simulink model "cruise_from_template"  (R2021a)
settings: Solver=ode3  StartTime=0.0  StopTime=60  FixedStep=1/120  RelTol=1e-5
model workspace (MATLAB code in the model file + MAT data in the model file):
  aeroCoeff.Cl0 = 0
  aeroCoeff.Cl_beta = -0.0325103964148
  aeroCoeff.Cl_da = -0.11683362461
  aeroCoeff.Cl_da_alpha = 0
  aeroCoeff.Cl_dr = 0.175731928031
  aeroCoeff.Cl_p = -0.836747044856
  aeroCoeff.Cl_r = 0.21079983888
  aeroCoeff.Cm0 = 0
  aeroCoeff.Cm_alpha = 2.67718247065
  aeroCoeff.Cm_alpha2 = 0
  aeroCoeff.Cm_beta2 = 0
  aeroCoeff.Cm_de = 2.06131250249
  aeroCoeff.Cm_df = 0
  aeroCoeff.Cm_q = -44.2196099405
  aeroCoeff.Cm_r = 0
  aeroCoeff.Cn0 = 0
  aeroCoeff.Cn_beta = 0.049110167229
  aeroCoeff.Cn_beta3 = 0
  aeroCoeff.Cn_da = 0.0191607144361
  aeroCoeff.Cn_dr = -0.388239776666
  aeroCoeff.Cn_p = -0.0358992823949
  aeroCoeff.Cn_q = 0.1595
  aeroCoeff.Cn_r = -0.0711145772129
  aeroCoeff.Cx0 = 0
  aeroCoeff.Cx_alpha = 0.609676812174
  aeroCoeff.Cx_alpha2 = 0
  aeroCoeff.Cx_alpha3 = 0
  aeroCoeff.Cx_df = 0
  aeroCoeff.Cx_df_alpha = 0
  aeroCoeff.Cx_dr = 0
  aeroCoeff.Cx_q = 0
  aeroCoeff.Cx_de = 0
  aeroCoeff.Cy0 = 0
  aeroCoeff.Cy_beta = -0.163321495037
  aeroCoeff.Cy_da = 0
  aeroCoeff.Cy_dr = 0.921751820421
  aeroCoeff.Cy_dr_alpha = 0
  aeroCoeff.Cy_p = -0.0243192462004
  aeroCoeff.Cy_r = 0.137581286748
  aeroCoeff.Cz0 = -0.82
  aeroCoeff.Cz_alpha = -3.9329056742
  aeroCoeff.Cz_alpha3 = 0
  aeroCoeff.Cz_de = -0.761136778285
  aeroCoeff.Cz_de_beta = 0
  aeroCoeff.Cz_df = 0
  aeroCoeff.Cz_df_alpha = 0
  aeroCoeff.Cz_q = 0.451102723983
  aeroCoeff.V0 = 64.72
  aeroCoeff.Cx_u = -0.223869966065
  aeroCoeff.Cz_u = -0.031521374419
  aeroCoeff.Cm_u = -0.00247698437476
  aeroCoeff.Cx_adot = 0
  aeroCoeff.Cz_adot = -5.62744914371
  aeroCoeff.Cm_adot = -19.0854006767
  environment.EarthRefAlt = 0
  initCond.x0 = [0 0 -1000]
  initCond.v0 = [64.72 0 0]
  initCond.euler0 = [0 0 0]
  initCond.w0 = [0 0 0]
  inputs0.time = 0
  inputs0.signals(1).dimensions = 1
  inputs0.signals(1).values = -0.104711430294
  inputs0.signals(2).dimensions = 1
  inputs0.signals(2).values = -0.0698725229544
  inputs0.signals(3).dimensions = 1
  inputs0.signals(3).values = -0.000215042330254
  states0.time = 0
  states0.signals(1).values = [0 0 -1000]
  states0.signals(1).dimensions = 3
  states0.signals(1).label = 'CSTATE'
  states0.signals(1).blockName = 'asb6DOFAirframeTemplate/6DOF EOM/6DOF (Euler Angles)/xe,ye,ze'
  states0.signals(1).stateName = ''
  states0.signals(1).inReferencedModel = 0
  states0.signals(1).sampleTime = [0 0]
  states0.signals(2).values = [0.128665353089 0.259337659946 -0.178947917154]
  states0.signals(2).dimensions = 3
  states0.signals(2).label = 'CSTATE'
  states0.signals(2).blockName = 'asb6DOFAirframeTemplate/6DOF EOM/6DOF (Euler Angles)/Calculate DCM &
    | Euler Angles/phi
    | theta
    | psi'
  states0.signals(2).stateName = ''
  states0.signals(2).inReferencedModel = 0
  states0.signals(2).sampleTime = [0 0]
  states0.signals(3).values = [36.9119692666 8.10720863264 8.82591882596]
  states0.signals(3).dimensions = 3
  states0.signals(3).label = 'CSTATE'
  states0.signals(3).blockName = 'asb6DOFAirframeTemplate/6DOF EOM/6DOF (Euler Angles)/ub,vb,wb'
  states0.signals(3).stateName = ''
  states0.signals(3).inReferencedModel = 0
  states0.signals(3).sampleTime = [0 0]
  states0.signals(4).values = [0 0 0]
  states0.signals(4).dimensions = 3
  states0.signals(4).label = 'CSTATE'
  states0.signals(4).blockName = 'asb6DOFAirframeTemplate/6DOF EOM/6DOF (Euler Angles)/p,q,r '
  states0.signals(4).stateName = ''
  states0.signals(4).inReferencedModel = 0
  states0.signals(4).sampleTime = [0 0]
  states0.signals(5).values = [0 0]
  states0.signals(5).dimensions = 2
  states0.signals(5).label = 'CSTATE'
  states0.signals(5).blockName = 'asb6DOFAirframeTemplate/Environment Model/Dryden Wind Turbulence Model 
    | (Continuous (+q +r))/Filters on velocities/Hwgw(s)/wg_p1'
  states0.signals(5).stateName = ''
  states0.signals(5).inReferencedModel = 0
  states0.signals(5).sampleTime = [0 0]
  states0.signals(6).values = [0 0]
  states0.signals(6).dimensions = 2
  states0.signals(6).label = 'CSTATE'
  states0.signals(6).blockName = 'asb6DOFAirframeTemplate/Environment Model/Dryden Wind Turbulence Model 
    | (Continuous (+q +r))/Filters on velocities/Hwgw(s)/wg_p2'
  states0.signals(6).stateName = ''
  states0.signals(6).inReferencedModel = 0
  states0.signals(6).sampleTime = [0 0]
  states0.signals(7).values = [0 0]
  states0.signals(7).dimensions = 2
  states0.signals(7).label = 'CSTATE'
  states0.signals(7).blockName = 'asb6DOFAirframeTemplate/Environment Model/Dryden Wind Turbulence Model 
    | (Continuous (+q +r))/Filters on velocities/Hvgw(s)/vg_p1'
  states0.signals(7).stateName = ''
  states0.signals(7).inReferencedModel = 0
  states0.signals(7).sampleTime = [0 0]
  states0.signals(8).values = [0 0]
  states0.signals(8).dimensions = 2
  states0.signals(8).label = 'CSTATE'
  states0.signals(8).blockName = 'asb6DOFAirframeTemplate/Environment Model/Dryden Wind Turbulence Model 
    | (Continuous (+q +r))/Filters on velocities/Hvgw(s)/vgw_p2'
  states0.signals(8).stateName = ''
  states0.signals(8).inReferencedModel = 0
  states0.signals(8).sampleTime = [0 0]
  states0.signals(9).values = [0 0]
  states0.signals(9).dimensions = 2
  states0.signals(9).label = 'CSTATE'
  states0.signals(9).blockName = 'asb6DOFAirframeTemplate/Environment Model/Dryden Wind Turbulence Model 
    | (Continuous (+q +r))/Filters on velocities/Hugw(s)/ug_p'
  states0.signals(9).stateName = ''
  states0.signals(9).inReferencedModel = 0
  states0.signals(9).sampleTime = [0 0]
  states0.signals(10).values = [0 0]
  states0.signals(10).dimensions = 2
  states0.signals(10).label = 'CSTATE'
  states0.signals(10).blockName = 'asb6DOFAirframeTemplate/Environment Model/Dryden Wind Turbulence Model 
    | (Continuous (+q +r))/Filters on angular rates/Hrgw/rgw_p'
  states0.signals(10).stateName = ''
  states0.signals(10).inReferencedModel = 0
  states0.signals(10).sampleTime = [0 0]
  states0.signals(11).values = [0 0]
  states0.signals(11).dimensions = 2
  states0.signals(11).label = 'CSTATE'
  states0.signals(11).blockName = 'asb6DOFAirframeTemplate/Environment Model/Dryden Wind Turbulence Model 
    | (Continuous (+q +r))/Filters on angular rates/Hqgw/qgw_p'
  states0.signals(11).stateName = ''
  states0.signals(11).inReferencedModel = 0
  states0.signals(11).sampleTime = [0 0]
  states0.signals(12).values = [0 0]
  states0.signals(12).dimensions = 2
  states0.signals(12).label = 'CSTATE'
  states0.signals(12).blockName = 'asb6DOFAirframeTemplate/Environment Model/Dryden Wind Turbulence Model 
    | (Continuous (+q +r))/Filters on angular rates/Hpgw/pgw_p'
  states0.signals(12).stateName = ''
  states0.signals(12).inReferencedModel = 0
  states0.signals(12).sampleTime = [0 0]
  vehicle.Sref = 16.834
  vehicle.cbar = 1.0141
  vehicle.bref = 8.704
  vehicle.CG = [0 0 0]
  vehicle.CP = [0 0 0]
  vehicle.inertia = [13609.1339893  0  146.582252166; 0  23776.5214  0; -146.582252166  0  34194.8393722]
  vehicle.acMass = 2950
  vehicle.Thrust = 2300
  vehicle.aileron_max = 0.523598775598
  vehicle.aileron_min = -0.523598775598
  vehicle.elevator_max = 0.305432619099
  vehicle.elevator_min = -0.305432619099
  vehicle.rudder_max = 0.436332312999
  vehicle.rudder_min = -0.436332312999
  other statements: initialize6DOFSkyHogg;
undefined symbols (not defined in the file): p, q, r
libraries: aerolibasang x3, shared6dof x1, aerolibadyn x1, aerolibatmos2 x1
settings Model: Creator=jakob  LastModifiedBy=jakob
settings SolverCC: AlgebraicLoopSolver=TrustRegion  AutoInsertRateTranBlk=on  InsertRTBMode=Never (minimum delay)  MinimalZcImpactIntegration=on
settings DataIOCC: ExternalInput=inputs0  InitialState=states0  SaveFormat=Array  SaveOutput=off
settings OptimizationCC: EnhancedBackFolding=on  StrengthReduction=on  InitFltsAndDblsToZero=on  DifferentSizesBufferReuse=on
settings DebuggingCC: WriteAfterWriteMsg=DisableAll  AlgebraicLoopMsg=none  FcnCallInpInsideContextMsg=warning  UnconnectedInputMsg=none  UnconnectedOutputMsg=none  UnconnectedLineMsg=none  UniqueDataStoreMsg=error  RootOutportRequireBusObject=none  StateNameClashWarn=warning  StrictBusMsg=ErrorOnBusTreatedAsVector  SFUnexpectedBacktrackingDiag=warning  SFNoUnconditionalDefaultTransitionDiag=warning  SFExecutionAtInitializationDiag=none  SFMachineParentedDataDiag=warning  ArithmeticOperatorsInVariantConditions=warning
settings ModelReferenceCC: PropagateSignalLabelsOutOfModel=off
settings SFSimCC: SimUseLocalCustomCode=off
settings RTWCC: RTWUseLocalCustomCode=off
settings CodeAppCC: StateflowObjectComments=on

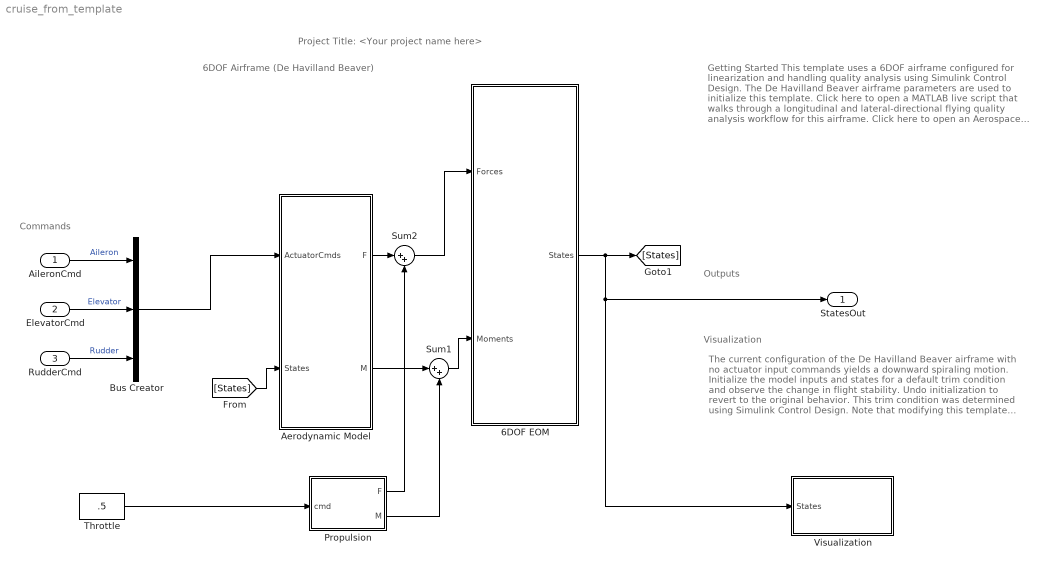
== system cruise_from_template ==
  note: Project Title: <Your project name here>
  note: 6DOF Airframe (De Havilland Beaver)
  note: Commands
  note: The current configuration of the De Havilland Beaver airframe with no actuator input commands yields a downward spiraling motion. Initialize the model inputs and states for a default trim condition and observe the change in flight stability. Undo initialization to revert to the original behavior. This trim condition was determined using Simulink Control Design. Note that modifying this template model may invalidate the default trim condition.
  note: Visualization
  note: Outputs
  note: Getting Started
      | This template uses a 6DOF airframe configured for linearization and handling quality analysis using Simulink Control Design. The De Havilland Beaver airframe parameters are used to initialize this template.
      |
      | Click here to open a MATLAB live script that walks through a longitudinal and lateral-directional flying quality analysis workflow for this airframe.
      |
      | Click here to open an Aerospace Blockset Flight Control Analysis template that can be customized to perform flying quality analysis on your airframe model.
  AileronCmd : Inport
  ElevatorCmd : Inport  Port=2
  RudderCmd : Inport  Port=3
  6DOF EOM : Subsystem  VariantControl=eom3DOF
  Aerodynamic Model : Subsystem  VariantControl=aeroCONST
  Bus Creator : BusCreator  Inputs=3
  Propulsion : Subsystem
      settings: RTWSystemCode=Inline
  Sum1 : Sum  Inputs=|++  InputSameDT=on  SaturateOnIntegerOverflow=on  OutDataTypeStr=Inherit: Same as first input
  Sum2 : Sum  Inputs=|++  InputSameDT=on  SaturateOnIntegerOverflow=on  OutDataTypeStr=Inherit: Same as first input
  Throttle : Constant  Value=.5
  Visualization : Subsystem
  StatesOut : Outport  OutDataTypeStr=double  VectorParamsAs1DForOutWhenUnconnected=off
  wires:
  AileronCmd/1 -> Bus Creator/1  "Aileron"
  ElevatorCmd/1 -> Bus Creator/2  "Elevator"
  RudderCmd/1 -> Bus Creator/3  "Rudder"
  [States] -> Aerodynamic Model/2(States)
  6DOF EOM/1(States) -> [States], StatesOut/1, Visualization/1(States)
  Sum2/1 -> 6DOF EOM/1(Forces)
  Propulsion/2(M) -> Sum1/2
  Propulsion/1(F) -> Sum2/2
  Throttle/1 -> Propulsion/1(cmd)
  Sum1/1 -> 6DOF EOM/2(Moments)
  Aerodynamic Model/1(F) -> Sum2/1
  Aerodynamic Model/2(M) -> Sum1/1
  Bus Creator/1 -> Aerodynamic Model/1(ActuatorCmds)

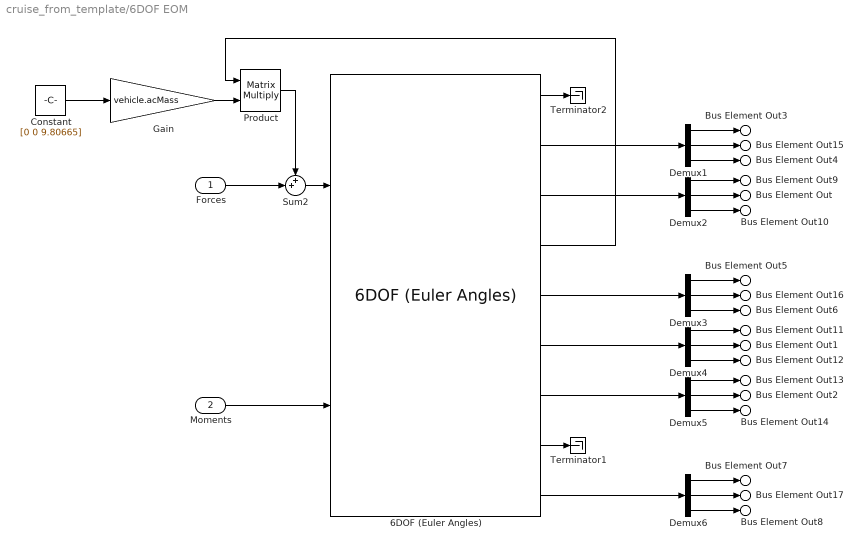
== system cruise_from_template/6DOF EOM ==
  Forces : Inport
  Moments : Inport  Port=2
  6DOF (Euler Angles) : shared6dof/6DOF (Euler Angles)  units=Metric (MKS)  mtype=Fixed  rep=Euler Angles  xme_0=initCond.x0  Vm_0=initCond.v0  eul_0=initCond.euler0  pm_0=initCond.w0  mass_0=vehicle.acMass  mass_e=0.5  mass_f=2.0  inertia=vehicle.inertia  inertia_e=eye(3)  inertia_f=2*eye(3)  k_quat=1.0  vre_flag=on  abi_flag=on  aMode=0  xme_statename={'Xe', 'Ye', 'Ze'}  Vm_statename={'Ubody', 'Vbody', 'Wbody'}  eul_statename={'phi', 'theta', 'psi'}  quat_statename={'qr', 'qi', 'qj','qk'}  pm_statename={'p', 'q', 'r'}  mass_statename=''
      settings: SourceProductBaseCode=AE,PW,DR,MT,UV,VE
  Constant : Constant  Value=[0 0 9.80665]
  Demux{1..6} (6 alike) : Demux  Outputs=3
  Gain : Gain  Gain=vehicle.acMass
  Product : Product  Multiplication=Matrix(*)
  Sum2 : Sum  Inputs=++|  InputSameDT=on  SaturateOnIntegerOverflow=on  OutDataTypeStr=Inherit: Same as first input
  Terminator1 : Terminator
  Terminator2 : Terminator
  Bus Element Out3 : Outport  VectorParamsAs1DForOutWhenUnconnected=off  PortName=States  Element=Xe
  Bus Element Out4 : Outport  VectorParamsAs1DForOutWhenUnconnected=off  PortName=States  Element=Ze
  Bus Element Out : Outport  VectorParamsAs1DForOutWhenUnconnected=off  PortName=States  Element=theta
  Bus Element Out5 : Outport  VectorParamsAs1DForOutWhenUnconnected=off  PortName=States  Element=u
  Bus Element Out6 : Outport  VectorParamsAs1DForOutWhenUnconnected=off  PortName=States  Element=w
  Bus Element Out1 : Outport  VectorParamsAs1DForOutWhenUnconnected=off  PortName=States  Element=q
  Bus Element Out2 : Outport  VectorParamsAs1DForOutWhenUnconnected=off  PortName=States  Element=q_dot
  Bus Element Out7 : Outport  VectorParamsAs1DForOutWhenUnconnected=off  PortName=States  Element=Axe
  Bus Element Out8 : Outport  VectorParamsAs1DForOutWhenUnconnected=off  PortName=States  Element=Aze
  Bus Element Out15 : Outport  VectorParamsAs1DForOutWhenUnconnected=off  PortName=States  Element=Ye
  Bus Element Out9 : Outport  VectorParamsAs1DForOutWhenUnconnected=off  PortName=States  Element=phi
  Bus Element Out10 : Outport  VectorParamsAs1DForOutWhenUnconnected=off  PortName=States  Element=psi
  Bus Element Out16 : Outport  VectorParamsAs1DForOutWhenUnconnected=off  PortName=States  Element=v
  Bus Element Out11 : Outport  VectorParamsAs1DForOutWhenUnconnected=off  PortName=States  Element=p
  Bus Element Out12 : Outport  VectorParamsAs1DForOutWhenUnconnected=off  PortName=States  Element=r
  Bus Element Out13 : Outport  VectorParamsAs1DForOutWhenUnconnected=off  PortName=States  Element=p_dot
  Bus Element Out14 : Outport  VectorParamsAs1DForOutWhenUnconnected=off  PortName=States  Element=r_dot
  Bus Element Out17 : Outport  VectorParamsAs1DForOutWhenUnconnected=off  PortName=States  Element=Aye
  wires:
  6DOF (Euler Angles)/2 -> Demux1/1
  6DOF (Euler Angles)/4 -> Product/1
  6DOF (Euler Angles)/1 -> Terminator2/1
  Demux6/2 -> Bus Element Out17/1
  Demux6/3 -> Bus Element Out8/1
  Demux6/1 -> Bus Element Out7/1
  6DOF (Euler Angles)/9 -> Demux6/1
  6DOF (Euler Angles)/7 -> Demux5/1
  Demux5/3 -> Bus Element Out14/1
  Demux5/2 -> Bus Element Out2/1
  Demux5/1 -> Bus Element Out13/1
  6DOF (Euler Angles)/6 -> Demux4/1
  Demux4/3 -> Bus Element Out12/1
  Demux4/2 -> Bus Element Out1/1
  Demux4/1 -> Bus Element Out11/1
  Demux3/3 -> Bus Element Out6/1
  Demux3/2 -> Bus Element Out16/1
  Demux3/1 -> Bus Element Out5/1
  6DOF (Euler Angles)/5 -> Demux3/1
  Demux2/3 -> Bus Element Out10/1
  Demux2/2 -> Bus Element Out/1
  Demux2/1 -> Bus Element Out9/1
  Demux1/1 -> Bus Element Out3/1
  Demux1/3 -> Bus Element Out4/1
  Demux1/2 -> Bus Element Out15/1
  Gain/1 -> Product/2
  6DOF (Euler Angles)/3 -> Demux2/1
  Moments/1 -> 6DOF (Euler Angles)/2
  Forces/1 -> Sum2/2
  Sum2/1 -> 6DOF (Euler Angles)/1
  Product/1 -> Sum2/1
  6DOF (Euler Angles)/8 -> Terminator1/1
  Constant/1 -> Gain/1

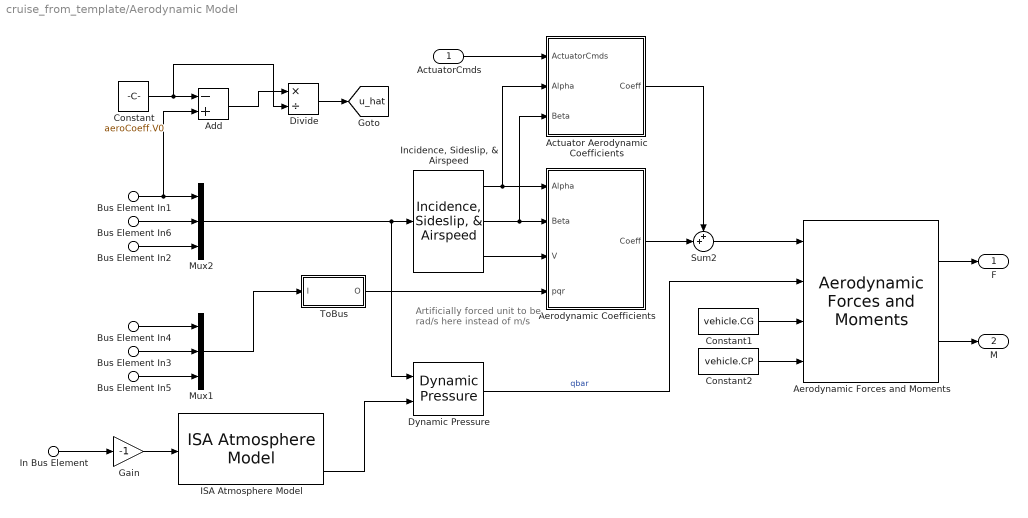
== system cruise_from_template/Aerodynamic Model ==
  note: Artificially forced unit to be
      | rad/s here instead of m/s
  ActuatorCmds : Inport
  Bus Element In1 : Inport  Port=2  PortName=States  Element=u
  Bus Element In2 : Inport  Port=2  PortName=States  Element=w
  Bus Element In3 : Inport  Port=2  PortName=States  Element=q
  Bus Element In6 : Inport  Port=2  PortName=States  Element=v
  Bus Element In4 : Inport  Port=2  PortName=States  Element=p
  Bus Element In5 : Inport  Port=2  PortName=States  Element=r
  In Bus Element : Inport  Port=2  PortName=States  Element=Ze
  Actuator Aerodynamic Coefficients : Subsystem
  Add : Sum  Inputs=-+
  Aerodynamic Coefficients : Subsystem
  Aerodynamic Forces and Moments : aerolibadyn/Aerodynamic Forces and Moments   inputAxes=Body  outputForceAxes=Body  outputMomentAxes=Body  S=vehicle.Sref  b=vehicle.bref  cbar=vehicle.cbar
  Constant : Constant  Value=aeroCoeff.V0
  Constant1 : Constant  Value=vehicle.CG
  Constant2 : Constant  Value=vehicle.CP
  Divide : Product  Inputs=*/
  Dynamic Pressure : aerolibasang/Dynamic Pressure
  Gain : Gain  Gain=-1
  ISA Atmosphere Model : aerolibatmos2/ISA Atmosphere Model  custom=off  g=9.80665  gamma=1.4  R=287.0531  L=0.0065  h_trop=11000  h_strat=20000  rho0=1.225  P0=101325  T0=288.15  h0=0
  "Incidence, Sideslip, & Airspeed" : aerolibasang/Incidence, Sideslip, & Airspeed
  Mux1 : Mux  Inputs=3
  Mux2 : Mux  Inputs=3
  Sum2 : Sum  Inputs=++|
  ToBus : Subsystem
  F : Outport  Unit=N  VectorParamsAs1DForOutWhenUnconnected=off
  M : Outport  Port=2  Unit=N*m  VectorParamsAs1DForOutWhenUnconnected=off
  tag scope: u_hat=global
  wires:
  ActuatorCmds/1 -> Actuator Aerodynamic Coefficients/1(ActuatorCmds)
  Bus Element In5/1 -> Mux1/3
  Bus Element In3/1 -> Mux1/2
  Bus Element In4/1 -> Mux1/1
  Actuator Aerodynamic Coefficients/1(Coeff) -> Sum2/1
  Aerodynamic Coefficients/1(Coeff) -> Sum2/2
  ToBus/1(O) -> Aerodynamic Coefficients/4(pqr)
  Mux2/1 -> Dynamic Pressure/1, "Incidence, Sideslip, & Airspeed"/1
  Dynamic Pressure/1 -> Aerodynamic Forces and Moments/2  "qbar"
  "Incidence, Sideslip, & Airspeed"/3 -> Aerodynamic Coefficients/3(V)
  "Incidence, Sideslip, & Airspeed"/2 -> Aerodynamic Coefficients/2(Beta), Actuator Aerodynamic Coefficients/3(Beta)
  Aerodynamic Forces and Moments/2 -> M/1
  Aerodynamic Forces and Moments/1 -> F/1
  Constant2/1 -> Aerodynamic Forces and Moments/4
  Constant1/1 -> Aerodynamic Forces and Moments/3
  Sum2/1 -> Aerodynamic Forces and Moments/1
  Bus Element In1/1 -> Add/2, Mux2/1
  Bus Element In6/1 -> Mux2/2
  Bus Element In2/1 -> Mux2/3
  "Incidence, Sideslip, & Airspeed"/1 -> Actuator Aerodynamic Coefficients/2(Alpha), Aerodynamic Coefficients/1(Alpha)
  Mux1/1 -> ToBus/1(I)
  ISA Atmosphere Model/4 -> Dynamic Pressure/2
  In Bus Element/1 -> Gain/1
  Gain/1 -> ISA Atmosphere Model/1
  Divide/1 -> [u_hat]
  Constant/1 -> Divide/2, Add/1
  Add/1 -> Divide/1

== system cruise_from_template/Propulsion ==
  cmd : Inport
  Mux : Mux  Inputs=[1 2]
  ThrustX : Lookup_n-D  NumberOfTableDimensions=1  LookupTableObject=''  BreakpointsForDimension1=(1/6)*(3+([-3:3]))  IndexSearchMethod=Linear search  BeginIndexSearchUsingPreviousIndexResult=on  Table=vehicle.Thrust*(1+tanh([-3:3]))  ExtrapMethod=Clip  InputSameDT=on
  ThrustYZ : Constant  Value=[0 0]'  SampleTime=-1
  Thrust_M1 : Constant  Value=[0 0 0]'  SampleTime=-1
  F : Outport  Unit=N  VectorParamsAs1DForOutWhenUnconnected=off
  M : Outport  Port=2  Unit=N*m  VectorParamsAs1DForOutWhenUnconnected=off
  wires:
  Thrust_M1/1 -> M/1
  ThrustX/1 -> Mux/1
  ThrustYZ/1 -> Mux/2
  Mux/1 -> F/1
  cmd/1 -> ThrustX/1

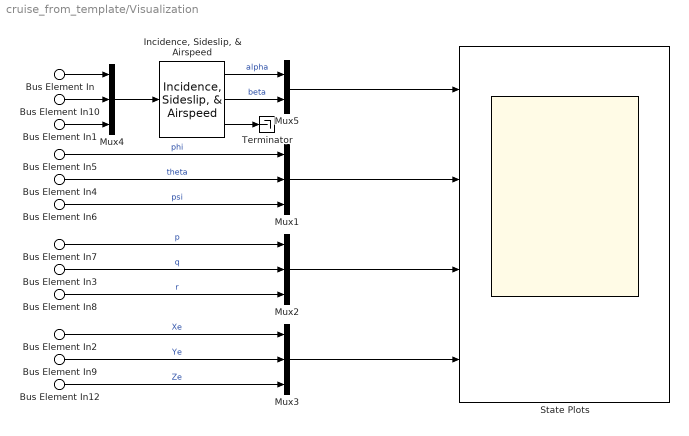
== system cruise_from_template/Visualization ==
  Bus Element In : Inport  PortName=States  Element=u
  Bus Element In1 : Inport  PortName=States  Element=w
  Bus Element In3 : Inport  PortName=States  Element=q
  Bus Element In4 : Inport  PortName=States  Element=theta
  Bus Element In12 : Inport  PortName=States  Element=Ze
  Bus Element In2 : Inport  PortName=States  Element=Xe
  Bus Element In10 : Inport  PortName=States  Element=v
  Bus Element In5 : Inport  PortName=States  Element=phi
  Bus Element In6 : Inport  PortName=States  Element=psi
  Bus Element In7 : Inport  PortName=States  Element=p
  Bus Element In8 : Inport  PortName=States  Element=r
  Bus Element In9 : Inport  PortName=States  Element=Ye
  "Incidence, Sideslip, & Airspeed" : aerolibasang/Incidence, Sideslip, & Airspeed
  Mux{1..4} (4 alike) : Mux  Inputs=3
  Mux5 : Mux  Inputs=2
  State Plots : Scope  NumInputPorts=4
  Terminator : Terminator
  wires:
  Mux3/1 -> State Plots/4
  Bus Element In2/1 -> Mux3/1  "Xe"
  Bus Element In9/1 -> Mux3/2  "Ye"
  Bus Element In12/1 -> Mux3/3  "Ze"
  Mux2/1 -> State Plots/3
  Mux1/1 -> State Plots/2
  Mux5/1 -> State Plots/1
  "Incidence, Sideslip, & Airspeed"/2 -> Mux5/2  "beta"
  "Incidence, Sideslip, & Airspeed"/1 -> Mux5/1  "alpha"
  Mux4/1 -> "Incidence, Sideslip, & Airspeed"/1
  Bus Element In10/1 -> Mux4/2
  Bus Element In8/1 -> Mux2/3  "r"
  Bus Element In7/1 -> Mux2/1  "p"
  Bus Element In6/1 -> Mux1/3  "psi"
  Bus Element In5/1 -> Mux1/1  "phi"
  Bus Element In4/1 -> Mux1/2  "theta"
  Bus Element In3/1 -> Mux2/2  "q"
  Bus Element In1/1 -> Mux4/3
  Bus Element In/1 -> Mux4/1
  "Incidence, Sideslip, & Airspeed"/3 -> Terminator/1

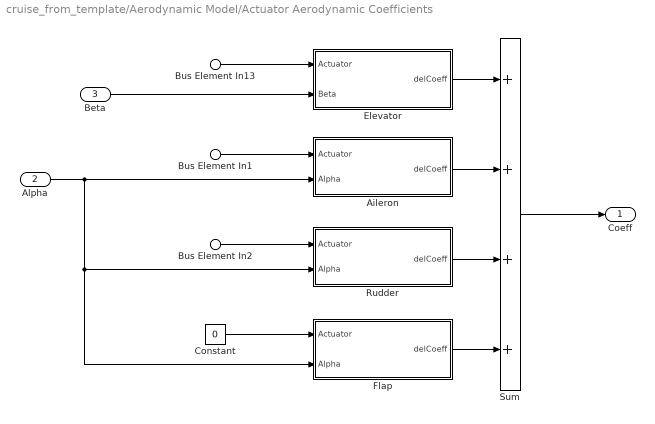
== system cruise_from_template/Aerodynamic Model/Actuator Aerodynamic Coefficients ==
  Bus Element In13 : Inport  PortName=ActuatorCmds  Element=Elevator
  Bus Element In1 : Inport  PortName=ActuatorCmds  Element=Aileron
  Bus Element In2 : Inport  PortName=ActuatorCmds  Element=Rudder
  Alpha : Inport  Port=2
  Beta : Inport  Port=3
  Aileron : Subsystem
  Constant : Constant  Value=0
  Elevator : Subsystem
  Flap : Subsystem
  Rudder : Subsystem
  Sum : Sum  Inputs=4  InputSameDT=on  SaturateOnIntegerOverflow=on  OutDataTypeStr=Inherit: Same as first input
  Coeff : Outport  InitialOutput=0  VectorParamsAs1DForOutWhenUnconnected=off
  wires:
  Constant/1 -> Flap/1(Actuator)
  Bus Element In2/1 -> Rudder/1(Actuator)
  Bus Element In1/1 -> Aileron/1(Actuator)
  Bus Element In13/1 -> Elevator/1(Actuator)
  Beta/1 -> Elevator/2(Beta)
  Flap/1(delCoeff) -> Sum/4
  Alpha/1 -> Flap/2(Alpha), Rudder/2(Alpha), Aileron/2(Alpha)
  Rudder/1(delCoeff) -> Sum/3
  Aileron/1(delCoeff) -> Sum/2
  Elevator/1(delCoeff) -> Sum/1
  Sum/1 -> Coeff/1

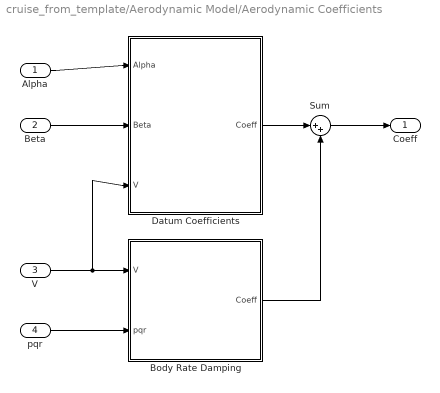
== system cruise_from_template/Aerodynamic Model/Aerodynamic Coefficients ==
  Alpha : Inport
  Beta : Inport  Port=2
  V : Inport  Port=3
  pqr : Inport  Port=4  Unit=rad/s
  Body Rate Damping : Subsystem
  Datum Coefficients : Subsystem
  Sum : Sum  Inputs=|++
  Coeff : Outport  VectorParamsAs1DForOutWhenUnconnected=off
  wires:
  pqr/1 -> Body Rate Damping/2(pqr)
  Sum/1 -> Coeff/1
  V/1 -> Datum Coefficients/3(V), Body Rate Damping/1(V)
  Body Rate Damping/1(Coeff) -> Sum/2
  Datum Coefficients/1(Coeff) -> Sum/1
  Beta/1 -> Datum Coefficients/2(Beta)
  Alpha/1 -> Datum Coefficients/1(Alpha)

== system cruise_from_template/Aerodynamic Model/ToBus ==
  I : Inport  Unit=rad/s
  Bus Creator3 : BusCreator  Inputs=p,q,r
  Demux : Demux  Outputs=3
  O : Outport  Unit=rad/s  VectorParamsAs1DForOutWhenUnconnected=off
  wires:
  I/1 -> Demux/1
  Demux/2 -> Bus Creator3/2  "q"
  Bus Creator3/1 -> O/1
  Demux/3 -> Bus Creator3/3  "r"
  Demux/1 -> Bus Creator3/1  "p"

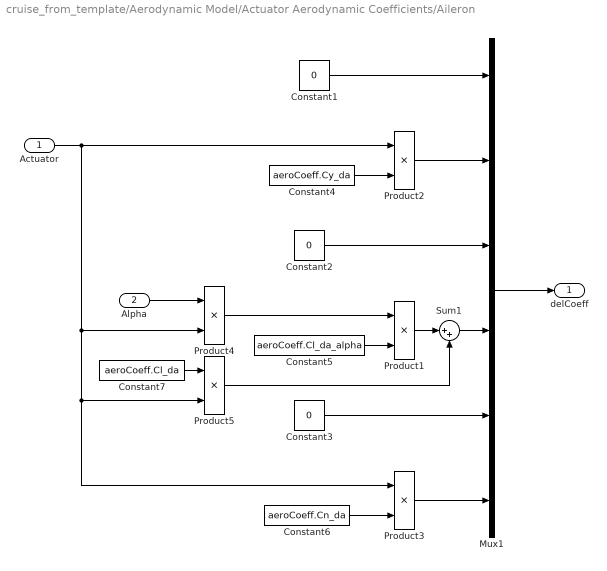
== system cruise_from_template/Aerodynamic Model/Actuator Aerodynamic Coefficients/Aileron ==
  Actuator : Inport
  Alpha : Inport  Port=2
  Constant1 : Constant  Value=0
  Constant2 : Constant  Value=0
  Constant3 : Constant  Value=0
  Constant4 : Constant  Value=aeroCoeff.Cy_da
  Constant5 : Constant  Value=aeroCoeff.Cl_da_alpha
  Constant6 : Constant  Value=aeroCoeff.Cn_da
  Constant7 : Constant  Value=aeroCoeff.Cl_da
  Mux1 : Mux  Inputs=6
  Product{1..5} (5 alike) : Product  InputSameDT=on  SaturateOnIntegerOverflow=on  OutDataTypeStr=Inherit: Same as first input
  Sum1 : Sum  Inputs=|++
  delCoeff : Outport  VectorParamsAs1DForOutWhenUnconnected=off
  wires:
  Product5/1 -> Sum1/2
  Constant7/1 -> Product5/1
  Sum1/1 -> Mux1/4
  Product4/1 -> Product1/1
  Alpha/1 -> Product4/1
  Constant6/1 -> Product3/2
  Product3/1 -> Mux1/6
  Actuator/1 -> Product2/1, Product3/1, Product5/2, Product4/2
  Product1/1 -> Sum1/1
  Constant5/1 -> Product1/2
  Constant4/1 -> Product2/2
  Constant3/1 -> Mux1/5
  Constant2/1 -> Mux1/3
  Constant1/1 -> Mux1/1
  Mux1/1 -> delCoeff/1
  Product2/1 -> Mux1/2

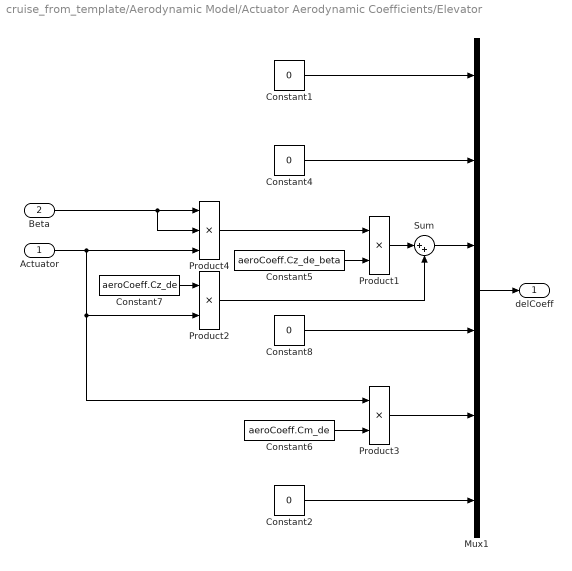
== system cruise_from_template/Aerodynamic Model/Actuator Aerodynamic Coefficients/Elevator ==
  Actuator : Inport
  Beta : Inport  Port=2
  Constant{1..2,4,8} (4 alike) : Constant  Value=0
  Constant5 : Constant  Value=aeroCoeff.Cz_de_beta
  Constant6 : Constant  Value=aeroCoeff.Cm_de
  Constant7 : Constant  Value=aeroCoeff.Cz_de
  Mux1 : Mux  Inputs=6
  Product1 : Product  InputSameDT=on  SaturateOnIntegerOverflow=on  OutDataTypeStr=Inherit: Same as first input
  Product2 : Product  InputSameDT=on  SaturateOnIntegerOverflow=on  OutDataTypeStr=Inherit: Same as first input
  Product3 : Product  InputSameDT=on  SaturateOnIntegerOverflow=on  OutDataTypeStr=Inherit: Same as first input
  Product4 : Product  Inputs=3  InputSameDT=on  SaturateOnIntegerOverflow=on  OutDataTypeStr=Inherit: Same as first input
  Sum : Sum  Inputs=|++
  delCoeff : Outport  VectorParamsAs1DForOutWhenUnconnected=off
  wires:
  Product2/1 -> Sum/2
  Beta/1 -> Product4/1, Product4/2
  Product3/1 -> Mux1/5
  Constant2/1 -> Mux1/6
  Constant8/1 -> Mux1/4
  Constant1/1 -> Mux1/1
  Product1/1 -> Sum/1
  Mux1/1 -> delCoeff/1
  Constant4/1 -> Mux1/2
  Constant7/1 -> Product2/1
  Product4/1 -> Product1/1
  Constant5/1 -> Product1/2
  Constant6/1 -> Product3/2
  Actuator/1 -> Product4/3, Product2/2, Product3/1
  Sum/1 -> Mux1/3

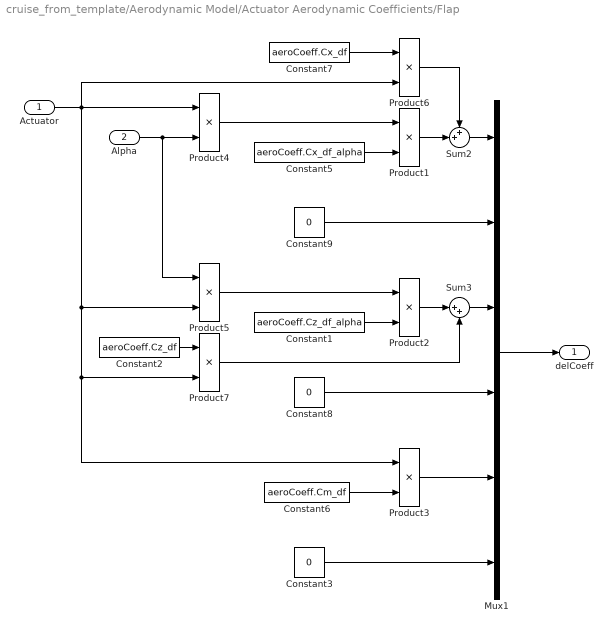
== system cruise_from_template/Aerodynamic Model/Actuator Aerodynamic Coefficients/Flap ==
  Actuator : Inport
  Alpha : Inport  Port=2
  Constant1 : Constant  Value=aeroCoeff.Cz_df_alpha
  Constant2 : Constant  Value=aeroCoeff.Cz_df
  Constant3 : Constant  Value=0
  Constant5 : Constant  Value=aeroCoeff.Cx_df_alpha
  Constant6 : Constant  Value=aeroCoeff.Cm_df
  Constant7 : Constant  Value=aeroCoeff.Cx_df
  Constant8 : Constant  Value=0
  Constant9 : Constant  Value=0
  Mux1 : Mux  Inputs=6
  Product{1..7} (7 alike) : Product  InputSameDT=on  SaturateOnIntegerOverflow=on  OutDataTypeStr=Inherit: Same as first input
  Sum2 : Sum  Inputs=++|
  Sum3 : Sum  Inputs=|++
  delCoeff : Outport  VectorParamsAs1DForOutWhenUnconnected=off
  wires:
  Product7/1 -> Sum3/2
  Product6/1 -> Sum2/1
  Product1/1 -> Sum2/2
  Constant1/1 -> Product2/2
  Product5/1 -> Product2/1
  Alpha/1 -> Product5/1, Product4/2
  Constant2/1 -> Product7/1
  Product2/1 -> Sum3/1
  Sum3/1 -> Mux1/3
  Sum2/1 -> Mux1/1
  Product3/1 -> Mux1/5
  Constant9/1 -> Mux1/2
  Constant8/1 -> Mux1/4
  Mux1/1 -> delCoeff/1
  Constant3/1 -> Mux1/6
  Constant7/1 -> Product6/1
  Product4/1 -> Product1/1
  Constant5/1 -> Product1/2
  Constant6/1 -> Product3/2
  Actuator/1 -> Product4/1, Product7/2, Product3/1, Product5/2, Product6/2

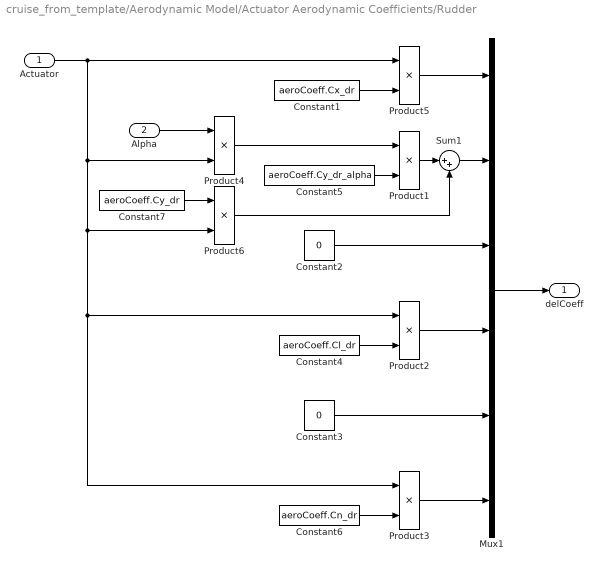
== system cruise_from_template/Aerodynamic Model/Actuator Aerodynamic Coefficients/Rudder ==
  Actuator : Inport
  Alpha : Inport  Port=2
  Constant1 : Constant  Value=aeroCoeff.Cx_dr
  Constant2 : Constant  Value=0
  Constant3 : Constant  Value=0
  Constant4 : Constant  Value=aeroCoeff.Cl_dr
  Constant5 : Constant  Value=aeroCoeff.Cy_dr_alpha
  Constant6 : Constant  Value=aeroCoeff.Cn_dr
  Constant7 : Constant  Value=aeroCoeff.Cy_dr
  Mux1 : Mux  Inputs=6
  Product{1..6} (6 alike) : Product  InputSameDT=on  SaturateOnIntegerOverflow=on  OutDataTypeStr=Inherit: Same as first input
  Sum1 : Sum  Inputs=|++
  delCoeff : Outport  VectorParamsAs1DForOutWhenUnconnected=off
  wires:
  Product6/1 -> Sum1/2
  Sum1/1 -> Mux1/2
  Product5/1 -> Mux1/1
  Constant1/1 -> Product5/2
  Product2/1 -> Mux1/4
  Product3/1 -> Mux1/6
  Constant4/1 -> Product2/2
  Product1/1 -> Sum1/1
  Mux1/1 -> delCoeff/1
  Constant3/1 -> Mux1/5
  Constant7/1 -> Product6/1
  Constant2/1 -> Mux1/3
  Alpha/1 -> Product4/1
  Product4/1 -> Product1/1
  Constant5/1 -> Product1/2
  Constant6/1 -> Product3/2
  Actuator/1 -> Product5/1, Product4/2, Product6/2, Product2/1, Product3/1

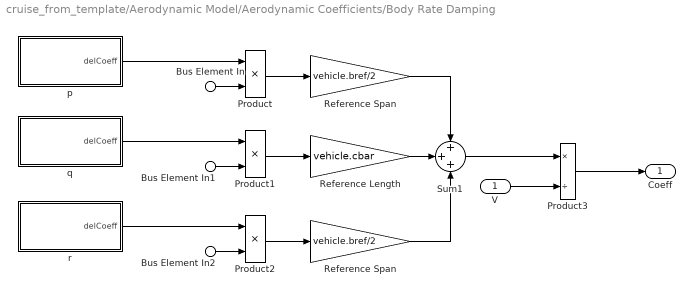
== system cruise_from_template/Aerodynamic Model/Aerodynamic Coefficients/Body Rate Damping ==
  V : Inport  Unit=m/s
  Bus Element In : Inport  Port=2  PortName=pqr  Element=p
  Bus Element In1 : Inport  Port=2  PortName=pqr  Element=q
  Bus Element In2 : Inport  Port=2  PortName=pqr  Element=r
  Product : Product  InputSameDT=on  SaturateOnIntegerOverflow=on  OutDataTypeStr=Inherit: Same as first input
  Product1 : Product  InputSameDT=on  SaturateOnIntegerOverflow=on  OutDataTypeStr=Inherit: Same as first input
  Product2 : Product  InputSameDT=on  SaturateOnIntegerOverflow=on  OutDataTypeStr=Inherit: Same as first input
  Product3 : Product  Inputs=*/  InputSameDT=on  SaturateOnIntegerOverflow=on  OutDataTypeStr=Inherit: Same as first input
  Reference Length : Gain  Gain=vehicle.cbar  SaturateOnIntegerOverflow=on  OutDataTypeStr=Inherit: Same as input  ParamDataTypeStr=Inherit: Same as input
  Reference Span : Gain  Gain=vehicle.bref/2  SaturateOnIntegerOverflow=on  OutDataTypeStr=Inherit: Same as input  ParamDataTypeStr=Inherit: Same as input
  "Reference Span " : Gain  Gain=vehicle.bref/2  SaturateOnIntegerOverflow=on  OutDataTypeStr=Inherit: Same as input  ParamDataTypeStr=Inherit: Same as input
  Sum1 : Sum  Inputs=+++  InputSameDT=on  SaturateOnIntegerOverflow=on  OutDataTypeStr=Inherit: Same as first input
  p : Subsystem
  q : Subsystem
  r : Subsystem
  Coeff : Outport  InitialOutput=0  VectorParamsAs1DForOutWhenUnconnected=off
  wires:
  Bus Element In/1 -> Product/2
  Bus Element In1/1 -> Product1/2
  Bus Element In2/1 -> Product2/2
  p/1(delCoeff) -> Product/1
  q/1(delCoeff) -> Product1/1
  Sum1/1 -> Product3/1
  V/1 -> Product3/2
  Product3/1 -> Coeff/1
  Product1/1 -> Reference Length/1
  Product2/1 -> "Reference Span "/1
  Product/1 -> Reference Span/1
  r/1(delCoeff) -> Product2/1
  Reference Length/1 -> Sum1/2
  Reference Span/1 -> Sum1/1
  "Reference Span "/1 -> Sum1/3

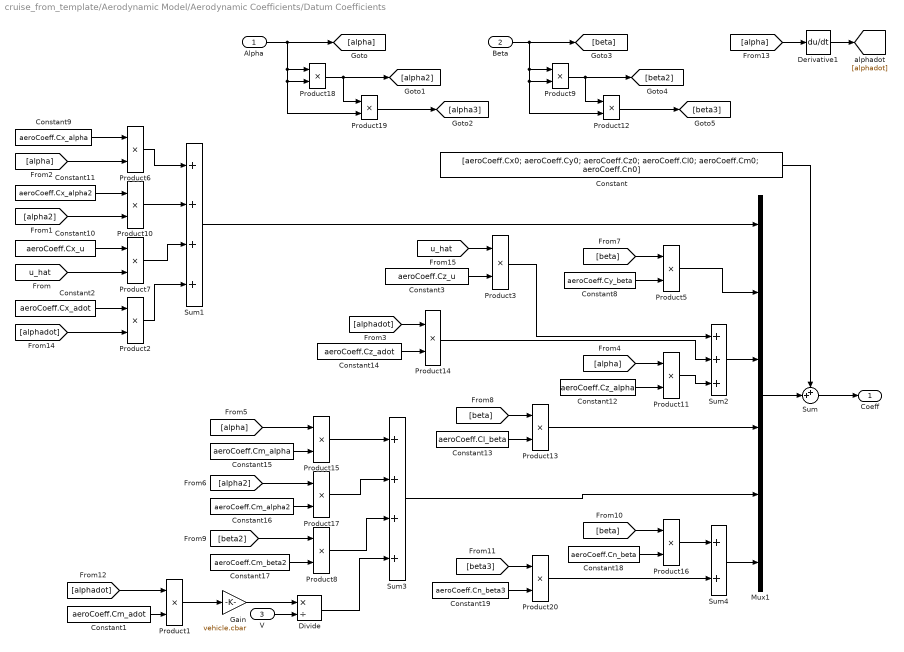
== system cruise_from_template/Aerodynamic Model/Aerodynamic Coefficients/Datum Coefficients ==
  Alpha : Inport
  Beta : Inport  Port=2
  V : Inport  Port=3
  Constant : Constant  Value=[aeroCoeff.Cx0; aeroCoeff.Cy0; aeroCoeff.Cz0; aeroCoeff.Cl0; aeroCoeff.Cm0; aeroCoeff.Cn0]
  Constant1 : Constant  Value=aeroCoeff.Cm_adot
  Constant10 : Constant  Value=aeroCoeff.Cx_u
  Constant11 : Constant  Value=aeroCoeff.Cx_alpha2
  Constant12 : Constant  Value=aeroCoeff.Cz_alpha
  Constant13 : Constant  Value=aeroCoeff.Cl_beta
  Constant14 : Constant  Value=aeroCoeff.Cz_adot
  Constant15 : Constant  Value=aeroCoeff.Cm_alpha
  Constant16 : Constant  Value=aeroCoeff.Cm_alpha2
  Constant17 : Constant  Value=aeroCoeff.Cm_beta2
  Constant18 : Constant  Value=aeroCoeff.Cn_beta
  Constant19 : Constant  Value=aeroCoeff.Cn_beta3
  Constant2 : Constant  Value=aeroCoeff.Cx_adot
  Constant3 : Constant  Value=aeroCoeff.Cz_u
  Constant8 : Constant  Value=aeroCoeff.Cy_beta
  Constant9 : Constant  Value=aeroCoeff.Cx_alpha
  Derivative1 : Derivative
  Divide : Product  Inputs=*/
  Gain : Gain  Gain=vehicle.cbar
  Mux1 : Mux  Inputs=6
  Product{1..3,5..20} (19 alike) : Product  InputSameDT=on  SaturateOnIntegerOverflow=on  OutDataTypeStr=Inherit: Same as first input
  Sum : Sum  Inputs=++|
  Sum1 : Sum  Inputs=++++  SaturateOnIntegerOverflow=on
  Sum2 : Sum  Inputs=3  SaturateOnIntegerOverflow=on
  Sum3 : Sum  Inputs=++++  SaturateOnIntegerOverflow=on
  Sum4 : Sum  Inputs=2  SaturateOnIntegerOverflow=on
  Coeff : Outport  InitialOutput=0  VectorParamsAs1DForOutWhenUnconnected=off
  wires:
  Sum/1 -> Coeff/1
  Constant/1 -> Sum/1
  Mux1/1 -> Sum/2
  Sum3/1 -> Mux1/5
  Product16/1 -> Sum4/1
  Product20/1 -> Sum4/2
  [beta3] -> Product20/1
  [beta] -> Product16/1
  Constant19/1 -> Product20/2
  Constant18/1 -> Product16/2
  Sum4/1 -> Mux1/6
  [beta2] -> Product8/1
  [beta] -> Product13/1
  [beta] -> Product5/1
  Beta/1 -> Product9/1, Product12/2, Product9/2, [beta]
  Product9/1 -> Product12/1, [beta2]
  Product12/1 -> [beta3]
  Product8/1 -> Sum3/3
  Constant17/1 -> Product8/2
  [alpha] -> Product15/1
  [alpha] -> Product11/1
  [alphadot] -> Product14/1
  [alpha] -> Product6/2
  [alpha2] -> Product10/2
  Constant10/1 -> Product7/1
  [u_hat] -> Product7/2
  Product19/1 -> [alpha3]
  Product18/1 -> [alpha2], Product19/1
  Alpha/1 -> [alpha], Product18/2, Product19/2, Product18/1
  Constant16/1 -> Product17/2
  Product17/1 -> Sum3/2
  [alpha2] -> Product17/1
  Constant15/1 -> Product15/2
  Product15/1 -> Sum3/1
  Constant14/1 -> Product14/2
  Product13/1 -> Mux1/4
  Constant13/1 -> Product13/2
  Sum2/1 -> Mux1/3
  Constant12/1 -> Product11/2
  Product10/1 -> Sum1/2
  Product6/1 -> Sum1/1
  Product7/1 -> Sum1/3
  Constant11/1 -> Product10/1
  Constant9/1 -> Product6/1
  Sum1/1 -> Mux1/1
  Product5/1 -> Mux1/2
  Constant8/1 -> Product5/2
  [alphadot] -> Product1/1
  Constant1/1 -> Product1/2
  Product1/1 -> Gain/1
  [alpha] -> Derivative1/1
  Derivative1/1 -> [alphadot]
  [alphadot] -> Product2/2
  Constant2/1 -> Product2/1
  Product2/1 -> Sum1/4
  Gain/1 -> Divide/1
  Divide/1 -> Sum3/4
  V/1 -> Divide/2
  Constant3/1 -> Product3/2
  [u_hat] -> Product3/1
  Product11/1 -> Sum2/3
  Product14/1 -> Sum2/2
  Product3/1 -> Sum2/1

== system cruise_from_template/Aerodynamic Model/Aerodynamic Coefficients/Body Rate Damping/p ==
  Constant1 : Constant  Value=0
  Constant2 : Constant  Value=0
  Constant3 : Constant  Value=0
  Constant4 : Constant  Value=aeroCoeff.Cl_p
  Constant5 : Constant  Value=aeroCoeff.Cn_p
  Constant8 : Constant  Value=aeroCoeff.Cy_p
  Mux1 : Mux  Inputs=6
  delCoeff : Outport  VectorParamsAs1DForOutWhenUnconnected=off
  wires:
  Constant4/1 -> Mux1/4
  Constant5/1 -> Mux1/6
  Constant8/1 -> Mux1/2
  Constant2/1 -> Mux1/3
  Constant3/1 -> Mux1/5
  Constant1/1 -> Mux1/1
  Mux1/1 -> delCoeff/1

== system cruise_from_template/Aerodynamic Model/Aerodynamic Coefficients/Body Rate Damping/q ==
  Constant1 : Constant  Value=0
  Constant2 : Constant  Value=0
  Constant3 : Constant  Value=aeroCoeff.Cn_q
  Constant4 : Constant  Value=aeroCoeff.Cz_q
  Constant5 : Constant  Value=aeroCoeff.Cm_q
  Constant8 : Constant  Value=aeroCoeff.Cx_q
  Mux1 : Mux  Inputs=6
  delCoeff : Outport  VectorParamsAs1DForOutWhenUnconnected=off
  wires:
  Constant3/1 -> Mux1/6
  Constant5/1 -> Mux1/5
  Constant4/1 -> Mux1/3
  Constant8/1 -> Mux1/1
  Constant1/1 -> Mux1/2
  Constant2/1 -> Mux1/4
  Mux1/1 -> delCoeff/1

== system cruise_from_template/Aerodynamic Model/Aerodynamic Coefficients/Body Rate Damping/r ==
  Constant1 : Constant  Value=0
  Constant2 : Constant  Value=0
  Constant3 : Constant  Value=aeroCoeff.Cm_r
  Constant4 : Constant  Value=aeroCoeff.Cl_r
  Constant5 : Constant  Value=aeroCoeff.Cn_r
  Constant6 : Constant  Value=aeroCoeff.Cy_r
  Mux1 : Mux  Inputs=6
  delCoeff : Outport  VectorParamsAs1DForOutWhenUnconnected=off
  wires:
  Constant6/1 -> Mux1/2
  Constant2/1 -> Mux1/3
  Constant3/1 -> Mux1/5
  Constant5/1 -> Mux1/6
  Constant1/1 -> Mux1/1
  Mux1/1 -> delCoeff/1
  Constant4/1 -> Mux1/4
